simulink model "Plant_test"  (R2026a)
settings: Solver=VariableStepAuto
values from neighbouring files (symbols this model uses):
  d_eq = abs(den_a(end-1) / num_a(end))    [main.m]
  J_eq = abs(den_a(end-2) / num_a(end))    [main.m]
  k_eq = delB.k_Nm_per_rad    [controller_design.m]    (also in main.m = abs(den_a(end)   / num_a(end)); nominal_plant_sizing.m = margin * Umax * r_arm * km / (R * theta_max))
  r_sensor = 0.052    [main.m]
  ts = 0.0005    [Hm_frd_deliverable_P.mat]    (also in deliverable_p_chirp.mat; frequency_response_initialization.m; main.m)
libraries: cstblocks_lti x2
settings Model: Creator=gicub  LastModifiedBy=aryan

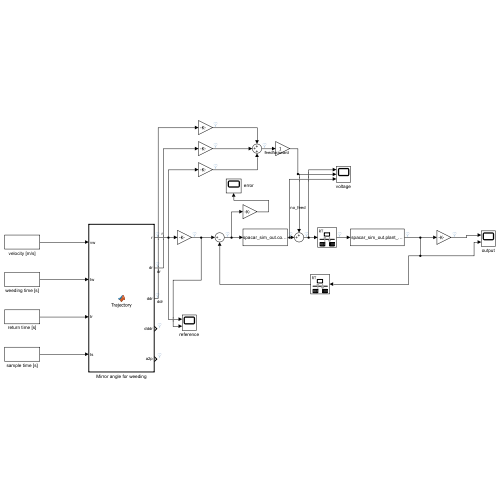
[thumbnail: Simulink's stored preview of the top-level diagram]
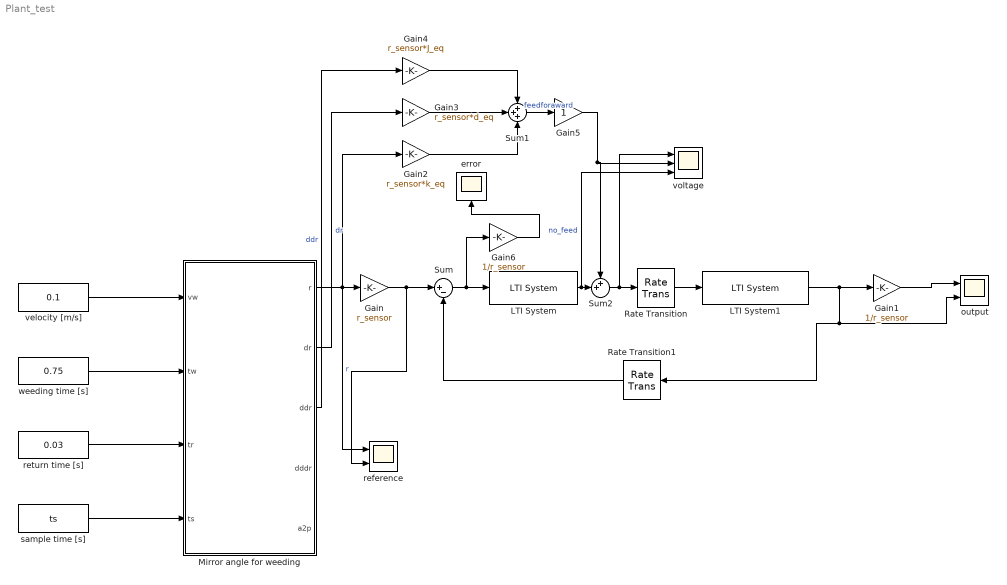
== system Plant_test ==
  Gain : Gain  Gain=r_sensor
  Gain1 : Gain  Gain=1/r_sensor
  Gain2 : Gain  Gain=r_sensor*k_eq
  Gain3 : Gain  Gain=r_sensor*d_eq
  Gain4 : Gain  Gain=r_sensor*J_eq
  Gain5 : Gain
  Gain6 : Gain  Gain=1/r_sensor
  LTI System : cstblocks_lti/LTI System  sys=spacar_sim_out.controller_retunedPID  IC=[]  PadeOrder=0
  LTI System1 : cstblocks_lti/LTI System  sys=spacar_sim_out.plant_voltage_to_sensor_reduced  IC=[]  PadeOrder=0
  Mirror angle for weeding : MATLAB Function  TreatAsAtomicUnit=on
  Rate Transition : RateTransition  Deterministic=off  OutPortSampleTimeOpt=Inherit
  Rate Transition1 : RateTransition  Deterministic=off  OutPortSampleTimeOpt=Inherit
  Sum : Sum  Inputs=|+-
  Sum1 : Sum  Inputs=+++
  Sum2 : Sum  Inputs=++|
  error : Scope
      settings: ActiveDisplayYMinimum=-0.00015521441150243072  ActiveDisplayYMaximum=0.00016263536321831844
  output : Scope  NumInputPorts=2
      settings: ActiveDisplayYMinimum=-0.02036  ActiveDisplayYMaximum=0.03432
  reference : Scope  NumInputPorts=2
      settings: ActiveDisplayYMinimum=-0.01957  ActiveDisplayYMaximum=0.01886
  return time [s] : Constant  Value=0.03  SampleTime=ts
  sample time [s] : Constant  Value=ts  SampleTime=ts
  velocity [m/s] : Constant  Value=0.1  SampleTime=ts
  voltage : Scope  NumInputPorts=3
      settings: ActiveDisplayYMinimum=-7.5601635211029432  ActiveDisplayYMaximum=5.818333907813944  DataLoggingVariableName=ScopeData2
  weeding time [s] : Constant  Value=0.75  SampleTime=ts
  wires:
  velocity [m/s]/1 -> Mirror angle for weeding/1(vw)
  return time [s]/1 -> Mirror angle for weeding/3(tr)
  weeding time [s]/1 -> Mirror angle for weeding/2(tw)
  sample time [s]/1 -> Mirror angle for weeding/4(ts)
  Mirror angle for weeding/1(r) -> Gain2/1, Gain/1, reference/1  "r"
  Sum/1 -> Gain6/1, LTI System/1
  Rate Transition/1 -> LTI System1/1
  LTI System1/1 -> Rate Transition1/1, output/2, Gain1/1
  Rate Transition1/1 -> Sum/2
  Gain1/1 -> output/1
  Gain/1 -> reference/2, Sum/1
  Mirror angle for weeding/2(dr) -> Gain3/1  "dr"
  Mirror angle for weeding/3(ddr) -> Gain4/1  "ddr"
  Gain3/1 -> Sum1/2
  Gain4/1 -> Sum1/1
  Gain2/1 -> Sum1/3
  LTI System/1 -> voltage/3, Sum2/2  "no_feed"
  Sum2/1 -> voltage/1, Rate Transition/1
  Sum1/1 -> Gain5/1  "feedforaward"
  Gain5/1 -> Sum2/1, voltage/2
  Gain6/1 -> error/1

== matlab function Plant_test/Mirror angle for weeding ==
  data: vw input; tw input; tr input; r output; dr output; ddr output; dddr output; ts input; a2p output
function [r, dr, ddr, dddr, a2p]   = Trajectory(vw, tw, tr, ts)
% Generates the mirror angle trajectory for weeding

% OUTPUTS:
% reference trajectory
% r:       [m]     position 
% dr:      [m/s]   velocity 
% ddr:     [m/s^2] acceleration
% dddr:    [m/s^3] jerk
% a2p:     [m]     angle to position transmission

% INPUTS
% vw:       [m/s]   driving velocity
% tw:       [s]     weeding time
% tr:       [s]     return time
% ts:       [s]     sample time

% define time 
persistent t
if isempty(t)
    t = 0;
end
% update time
t = mod(t+ts,tw+tr);  % [s] time
at = 2*pi/tr*t;       % [1/s] angle in period

% auxiliary variables
D = vw*(tw+tr);    % [m] maximum spot amplitude
xs = (D*tw)/(2*(tr + tw)) + (D*(1 - tw^2/(tr + tw)^2)^(1/2))/(2*pi) - (D*tw*acos(tw/(tr + tw)))/(2*pi*(tr + tw)); % [m] maximum amplitude
a2p = xs/17.5e-3;  % [m] angle to position transmission
Da = D/a2p;        % [rad] angular amplitude
va = vw/a2p;       % [rad/s] angular velocity

a = Da*tw/(tw+tr)/2; % [m] polynomial offset cofficient
b = -2*a/tr;         % [m/s] polynomial slope coefficient
c = Da/(2*pi);       % [m] sinusoidal amplitude

% compute angular trajectory and time derivatives
if t <= tr
    % sinusoidal return part
    r       = a+b*t+c*sin(at);
    dr      = b + c*2*pi/tr*cos(at);
    ddr     = -c*(2*pi/tr)^2*sin(at);
    dddr    = -c*(2*pi/tr)^3*cos(at);
else
    % constant velocity welding part
    r       = -Da*tw/(tw+tr)/2+(t-tr)*va;
    dr      = va;
    ddr     = 0;
    dddr    = 0;
end
